simulink model "Quadruped_modelling"  (R2023b)
settings: Solver=VariableStepAuto  StartTime=0.0  StopTime=2.6  RelTol=1e-3
InitFcn:
  | robotParameters
undefined symbols (not defined in the file): foot_x, foot_y, foot_z, lower_leg_length, plane_x, plane_y, plane_z, torso_height, torso_length, torso_width, upper_leg_length, X, Y, Z
libraries: sm_lib x311, nesl_utility x41, walkingRobotUtils x4, sharedtransform x1
(part 9 of 9)

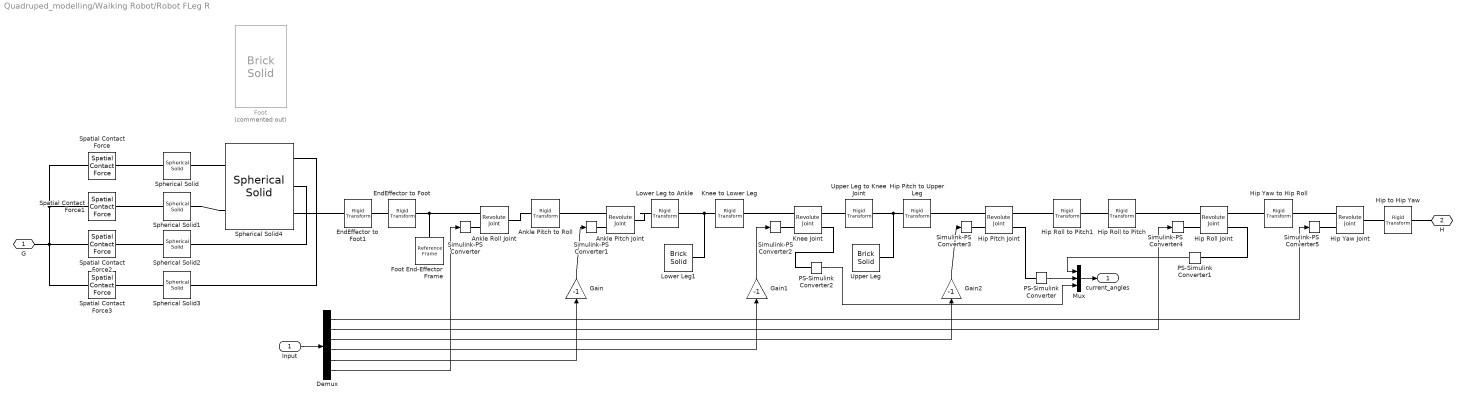
== system Quadruped_modelling/Walking Robot/Robot FLeg R ==
  Input : Inport
  Ankle Pitch Joint : sm_lib/Joints/Revolute Joint  JointMode=Normal  SenseConstraintForce=off  SenseConstraintForceX=off  SenseConstraintForceY=off  SenseConstraintForceZ=off  SenseConstraintTorque=off  SenseConstraintTorqueX=off  SenseConstraintTorqueY=off  SenseConstraintTorqueZ=off  SenseTotalForce=off  SenseTotalForceX=off  SenseTotalForceY=off  SenseTotalForceZ=off  SenseTotalTorque=off  SenseTotalTorqueX=off  SenseTotalTorqueY=off  SenseTotalTorqueZ=off  CompositeWrenchDir=FollowerOnBase  CompositeWrenchFrame=BaseFrame  EquilibriumPosition=0  EquilibriumPositionUnits=deg  SpringStiffness=0  SpringStiffnessUnits=N*m/deg  DampingCoefficient=1  DampingCoefficientUnits=N*m/(rad/s)  TorqueActuationMode=ComputedTorque  MotionActuationMode=InputMotion  SensePosition=off  SenseVelocity=off  SenseAcceleration=off  SenseTorqueForce=off  SenseLowerLimitTorqueForce=off  SenseUpperLimitTorqueForce=off  LowerLimitSpecify=on  LowerLimitBound=-pi/2  LowerLimitBoundUnits=rad  LowerLimitStiffness=100  LowerLimitStiffnessUnits=N*m/rad  LowerLimitDamping=10  LowerLimitDampingUnits=N*m/(rad/s)  LowerLimitTransitionRegionWidth=0.1  LowerLimitTransitionRegionWidthUnits=deg  UpperLimitSpecify=on  UpperLimitBound=pi/2  UpperLimitBoundUnits=rad  UpperLimitStiffness=100  UpperLimitStiffnessUnits=N*m/rad  UpperLimitDamping=10  UpperLimitDampingUnits=N*m/(rad/s)  UpperLimitTransitionRegionWidth=0.1  UpperLimitTransitionRegionWidthUnits=deg  PositionTargetSpecify=on  PositionTargetPriority=High  PositionTargetValue=0  PositionTargetValueUnits=rad  VelocityTargetSpecify=off  VelocityTargetPriority=High  VelocityTargetValue=0  VelocityTargetValueUnits=deg/s
  Ankle Pitch to Roll : sm_lib/Frames and Transforms/Rigid Transform  TranslationMethod=None  TranslationStandardOffset=0  TranslationStandardOffsetUnits=cm  TranslationStandardAxis=+Z  TranslationCartesianOffset=[0 0 upper_leg_length/2]  TranslationCartesianOffsetUnits=cm  TranslationROffset=0  TranslationROffsetUnits=m  TranslationZOffset=0  TranslationZOffsetUnits=m  TranslationThetaOffset=0  TranslationThetaOffsetUnits=deg  RotationMethod=StandardAxis  RotationAngleUnits=deg  RotationStandardAxis=+X  RotationAngle=90  RotationArbitraryAxis=[0 0 1]  FollAlignAxisA=+X  BaseAlignAxisA=+Y  FollAlignAxisB=+Y  BaseAlignAxisB=+Z  RotationSequenceAxes=FollowerAxes  RotationSequence=XYX  RotationSequenceAngles=[0 0 0]  RotationSequenceAnglesUnits=deg  RotationMatrix=[1 0 0; 0 1 0; 0 0 1]  Quaternion=[1 0 0 0]
  Ankle Roll Joint : sm_lib/Joints/Revolute Joint  JointMode=Normal  SenseConstraintForce=off  SenseConstraintForceX=off  SenseConstraintForceY=off  SenseConstraintForceZ=off  SenseConstraintTorque=off  SenseConstraintTorqueX=off  SenseConstraintTorqueY=off  SenseConstraintTorqueZ=off  SenseTotalForce=off  SenseTotalForceX=off  SenseTotalForceY=off  SenseTotalForceZ=off  SenseTotalTorque=off  SenseTotalTorqueX=off  SenseTotalTorqueY=off  SenseTotalTorqueZ=off  CompositeWrenchDir=FollowerOnBase  CompositeWrenchFrame=BaseFrame  EquilibriumPosition=0  EquilibriumPositionUnits=deg  SpringStiffness=0  SpringStiffnessUnits=N*m/deg  DampingCoefficient=1  DampingCoefficientUnits=N*m/(rad/s)  TorqueActuationMode=ComputedTorque  MotionActuationMode=InputMotion  SensePosition=off  SenseVelocity=off  SenseAcceleration=off  SenseTorqueForce=off  SenseLowerLimitTorqueForce=off  SenseUpperLimitTorqueForce=off  LowerLimitSpecify=on  LowerLimitBound=-pi/2  LowerLimitBoundUnits=rad  LowerLimitStiffness=100  LowerLimitStiffnessUnits=N*m/rad  LowerLimitDamping=10  LowerLimitDampingUnits=N*m/(rad/s)  LowerLimitTransitionRegionWidth=0.1  LowerLimitTransitionRegionWidthUnits=deg  UpperLimitSpecify=on  UpperLimitBound=pi/2  UpperLimitBoundUnits=rad  UpperLimitStiffness=100  UpperLimitStiffnessUnits=N*m/rad  UpperLimitDamping=10  UpperLimitDampingUnits=N*m/(rad/s)  UpperLimitTransitionRegionWidth=0.1  UpperLimitTransitionRegionWidthUnits=deg  PositionTargetSpecify=on  PositionTargetPriority=High  PositionTargetValue=0  PositionTargetValueUnits=rad  VelocityTargetSpecify=off  VelocityTargetPriority=High  VelocityTargetValue=0  VelocityTargetValueUnits=deg/s
  Demux : Demux  Outputs=6
  EndEffector to Foot : sm_lib/Frames and Transforms/Rigid Transform  TranslationMethod=None  TranslationStandardOffset=0  TranslationStandardOffsetUnits=cm  TranslationStandardAxis=+Z  TranslationCartesianOffset=[0 0 upper_leg_length/2]  TranslationCartesianOffsetUnits=cm  TranslationROffset=0  TranslationROffsetUnits=m  TranslationZOffset=0  TranslationZOffsetUnits=m  TranslationThetaOffset=0  TranslationThetaOffsetUnits=deg  RotationMethod=StandardAxis  RotationAngleUnits=deg  RotationStandardAxis=+Z  RotationAngle=-90  RotationArbitraryAxis=[0 0 1]  FollAlignAxisA=+X  BaseAlignAxisA=+Y  FollAlignAxisB=+Y  BaseAlignAxisB=+Z  RotationSequenceAxes=FollowerAxes  RotationSequence=XYX  RotationSequenceAngles=[0 0 0]  RotationSequenceAnglesUnits=deg  RotationMatrix=[1 0 0; 0 1 0; 0 0 1]  Quaternion=[1 0 0 0]
  EndEffector to Foot1 : sm_lib/Frames and Transforms/Rigid Transform  TranslationMethod=None  TranslationStandardOffset=0  TranslationStandardOffsetUnits=cm  TranslationStandardAxis=+Z  TranslationCartesianOffset=[0 0 upper_leg_length/2]  TranslationCartesianOffsetUnits=cm  TranslationROffset=0  TranslationROffsetUnits=m  TranslationZOffset=0  TranslationZOffsetUnits=m  TranslationThetaOffset=0  TranslationThetaOffsetUnits=deg  RotationMethod=StandardAxis  RotationAngleUnits=deg  RotationStandardAxis=+X  RotationAngle=180  RotationArbitraryAxis=[0 0 1]  FollAlignAxisA=+X  BaseAlignAxisA=+Y  FollAlignAxisB=+Y  BaseAlignAxisB=+Z  RotationSequenceAxes=FollowerAxes  RotationSequence=XYX  RotationSequenceAngles=[0 0 0]  RotationSequenceAnglesUnits=deg  RotationMatrix=[1 0 0; 0 1 0; 0 0 1]  Quaternion=[1 0 0 0]
  Foot : sm_lib/Body Elements/Brick Solid  Commented=on  GraphicAmbientColor=[0.15 0.15 0.15 1.0]  BasedOnType=Density  BrickDimensions=[foot_x foot_y foot_z]  BrickDimensionsUnits=m  CenterOfMass=[0 0 0]  CenterOfMassUnits=m  GraphicDiffuseColor=[0.5 0.5 0.5]  Density=200  DensityUnits=kg/(m^3)  DoExposeReferenceFrame=off  GraphicEmissiveColor=[0.0 0.0 0.0 1.0]  ExportEntireGeometry=off  SerializedFrames=<Frames><Frame><Id>Frame1</Id><Value><Name>F1</Name><Origin><Source>GeometricFeature</Source><FeatureName>+x -y curve</FeatureName></Origin><PrimaryAxis><DefinedDirection>+Z</DefinedDirection><Source>ReferenceFrame</Source><SourceDirection>+Z</SourceDirection><FeatureName></FeatureName></PrimaryAxis><SecondaryAxis><DefinedDirection>+X</DefinedDirection><Source>ReferenceFrame</Source><SourceDirection>+X</SourceDirection><FeatureName></FeatureName></SecondaryAxis></Value></Frame><Frame><Id>Frame2</Id><Value><Name>F2</Name><Origin><Source>GeometricFeature</Source><FeatureName>+x +y curve</FeatureName></Origin><PrimaryAxis><DefinedDirection>+Z</DefinedDirection><Source>ReferenceFrame</Source><SourceDirection>+Z</SourceDirection><FeatureName></FeatureName></PrimaryAxis><SecondaryAxis><DefinedDirection>+X</DefinedDirection><Source>ReferenceFrame</Source><SourceDirection>+X</SourceDirection><FeatureName></FeatureName></SecondaryAxis></Value></Frame><Frame><Id>Frame3</Id><Value><Name>F3</Name><Origin><Source>GeometricFeature</Source><FeatureName>-x -y curve</FeatureName></Origin><PrimaryAxis><DefinedDirection>+Z</DefinedDirection><Source>ReferenceFrame</Source><SourceDirection>+Z</SourceDirection><FeatureName></FeatureName></PrimaryAxis><SecondaryAxis><DefinedDirection>+X</DefinedDirection><Source>ReferenceFrame</Source><SourceDirection>+X</SourceDirection><FeatureName></FeatureName></SecondaryAxis></Value></Frame><Frame><Id>Frame4</Id><Value><Name>F4</Name><Origin><Source>GeometricFeature</Source><FeatureName>-x +y curve</FeatureName></Origin><PrimaryAxis><DefinedDirection>+Z</DefinedDirection><Source>ReferenceFrame</Source><SourceDirection>+Z</SourceDirection><FeatureName></FeatureName></PrimaryAxis><SecondaryAxis><DefinedDirection>+X</DefinedDirection><Source>ReferenceFrame</Source><SourceDirection>+X</SourceDirection><FeatureName></FeatureName></SecondaryAxis></Value></Frame><Frame><Id>Frame5</Id><Value><Name>A</Name><Origin><Source>GeometricFeature</Source><FeatureName>+z surface</FeatureName></Origin><PrimaryAxis><DefinedDirection>+Z</DefinedDirection><Source>ReferenceFrame</Source><SourceDirection>-Y</SourceDirection><FeatureName></FeatureName></PrimaryAxis><SecondaryAxis><DefinedDirection>+X</DefinedDirection><Source>ReferenceFrame</Source><SourceDirection>+X</SourceDirection><FeatureName></FeatureName></SecondaryAxis></Value></Frame></Frames>  MarkerShape=Sphere  MarkerSize=10  GraphicType=FromGeometry  InertiaType=CalculateFromGeometry  Mass=1  MassUnits=kg  MomentsOfInertia=[1 1 1]  MomentsOfInertiaUnits=kg*m^2  GraphicOpacity=1.0  ProductsOfInertia=[0 0 0]  ProductsOfInertiaUnits=kg*m^2  GraphicShininess=75  GraphicSpecularColor=[0.5 0.5 0.5 1.0]  GraphicVisPropType=SimpleVisualProperties
  Foot End-Effector Frame : sm_lib/Frames and Transforms/Reference Frame
  Gain : Gain  Gain=-1
  Gain1 : Gain  Gain=-1
  Gain2 : Gain  Gain=-1
  Hip Pitch Joint : sm_lib/Joints/Revolute Joint  JointMode=Normal  SenseConstraintForce=off  SenseConstraintForceX=off  SenseConstraintForceY=off  SenseConstraintForceZ=off  SenseConstraintTorque=off  SenseConstraintTorqueX=off  SenseConstraintTorqueY=off  SenseConstraintTorqueZ=off  SenseTotalForce=off  SenseTotalForceX=off  SenseTotalForceY=off  SenseTotalForceZ=off  SenseTotalTorque=off  SenseTotalTorqueX=off  SenseTotalTorqueY=off  SenseTotalTorqueZ=off  CompositeWrenchDir=FollowerOnBase  CompositeWrenchFrame=BaseFrame  EquilibriumPosition=0  EquilibriumPositionUnits=deg  SpringStiffness=0  SpringStiffnessUnits=N*m/deg  DampingCoefficient=1  DampingCoefficientUnits=N*m/(rad/s)  TorqueActuationMode=ComputedTorque  MotionActuationMode=InputMotion  SensePosition=on  SenseVelocity=off  SenseAcceleration=off  SenseTorqueForce=off  SenseLowerLimitTorqueForce=off  SenseUpperLimitTorqueForce=off  LowerLimitSpecify=on  LowerLimitBound=-pi/2  LowerLimitBoundUnits=rad  LowerLimitStiffness=100  LowerLimitStiffnessUnits=N*m/rad  LowerLimitDamping=10  LowerLimitDampingUnits=N*m/(rad/s)  LowerLimitTransitionRegionWidth=0.1  LowerLimitTransitionRegionWidthUnits=deg  UpperLimitSpecify=on  UpperLimitBound=pi/2  UpperLimitBoundUnits=rad  UpperLimitStiffness=100  UpperLimitStiffnessUnits=N*m/rad  UpperLimitDamping=10  UpperLimitDampingUnits=N*m/(rad/s)  UpperLimitTransitionRegionWidth=0.1  UpperLimitTransitionRegionWidthUnits=deg  PositionTargetSpecify=on  PositionTargetPriority=High  PositionTargetValue=0  PositionTargetValueUnits=rad  VelocityTargetSpecify=off  VelocityTargetPriority=High  VelocityTargetValue=0  VelocityTargetValueUnits=deg/s
  Hip Pitch to Upper Leg : sm_lib/Frames and Transforms/Rigid Transform  TranslationMethod=StandardAxis  TranslationStandardOffset=upper_leg_length/2  TranslationStandardOffsetUnits=m  TranslationStandardAxis=+X  TranslationCartesianOffset=[upper_leg_length/2 0 0]  TranslationCartesianOffsetUnits=m  TranslationROffset=0  TranslationROffsetUnits=m  TranslationZOffset=0  TranslationZOffsetUnits=m  TranslationThetaOffset=0  TranslationThetaOffsetUnits=deg  RotationMethod=StandardAxis  RotationAngleUnits=deg  RotationStandardAxis=+Y  RotationAngle=90  RotationArbitraryAxis=[0 0 1]  FollAlignAxisA=+X  BaseAlignAxisA=+Y  FollAlignAxisB=+Y  BaseAlignAxisB=+Z  RotationSequenceAxes=FollowerAxes  RotationSequence=XYX  RotationSequenceAngles=[0 0 0]  RotationSequenceAnglesUnits=deg  RotationMatrix=[1 0 0; 0 1 0; 0 0 1]  Quaternion=[1 0 0 0]
  Hip Roll Joint : sm_lib/Joints/Revolute Joint  JointMode=Normal  SenseConstraintForce=off  SenseConstraintForceX=off  SenseConstraintForceY=off  SenseConstraintForceZ=off  SenseConstraintTorque=off  SenseConstraintTorqueX=off  SenseConstraintTorqueY=off  SenseConstraintTorqueZ=off  SenseTotalForce=off  SenseTotalForceX=off  SenseTotalForceY=off  SenseTotalForceZ=off  SenseTotalTorque=off  SenseTotalTorqueX=off  SenseTotalTorqueY=off  SenseTotalTorqueZ=off  CompositeWrenchDir=FollowerOnBase  CompositeWrenchFrame=BaseFrame  EquilibriumPosition=0  EquilibriumPositionUnits=deg  SpringStiffness=0  SpringStiffnessUnits=N*m/deg  DampingCoefficient=1  DampingCoefficientUnits=N*m/(rad/s)  TorqueActuationMode=ComputedTorque  MotionActuationMode=InputMotion  SensePosition=on  SenseVelocity=off  SenseAcceleration=off  SenseTorqueForce=off  SenseLowerLimitTorqueForce=off  SenseUpperLimitTorqueForce=off  LowerLimitSpecify=on  LowerLimitBound=-pi/2  LowerLimitBoundUnits=rad  LowerLimitStiffness=100  LowerLimitStiffnessUnits=N*m/rad  LowerLimitDamping=10  LowerLimitDampingUnits=N*m/(rad/s)  LowerLimitTransitionRegionWidth=0.1  LowerLimitTransitionRegionWidthUnits=deg  UpperLimitSpecify=on  UpperLimitBound=pi/2  UpperLimitBoundUnits=rad  UpperLimitStiffness=100  UpperLimitStiffnessUnits=N*m/rad  UpperLimitDamping=10  UpperLimitDampingUnits=N*m/(rad/s)  UpperLimitTransitionRegionWidth=0.1  UpperLimitTransitionRegionWidthUnits=deg  PositionTargetSpecify=on  PositionTargetPriority=High  PositionTargetValue=0  PositionTargetValueUnits=rad  VelocityTargetSpecify=off  VelocityTargetPriority=High  VelocityTargetValue=0  VelocityTargetValueUnits=deg/s
  Hip Roll to Pitch : sm_lib/Frames and Transforms/Rigid Transform  TranslationMethod=None  TranslationStandardOffset=0  TranslationStandardOffsetUnits=cm  TranslationStandardAxis=+Z  TranslationCartesianOffset=[0 0 upper_leg_length/2]  TranslationCartesianOffsetUnits=cm  TranslationROffset=0  TranslationROffsetUnits=m  TranslationZOffset=0  TranslationZOffsetUnits=m  TranslationThetaOffset=0  TranslationThetaOffsetUnits=deg  RotationMethod=StandardAxis  RotationAngleUnits=deg  RotationStandardAxis=+Z  RotationAngle=-90  RotationArbitraryAxis=[0 0 1]  FollAlignAxisA=+X  BaseAlignAxisA=+Y  FollAlignAxisB=+Y  BaseAlignAxisB=+Z  RotationSequenceAxes=FollowerAxes  RotationSequence=XYX  RotationSequenceAngles=[0 0 0]  RotationSequenceAnglesUnits=deg  RotationMatrix=[1 0 0; 0 1 0; 0 0 1]  Quaternion=[1 0 0 0]
  Hip Roll to Pitch1 : sm_lib/Frames and Transforms/Rigid Transform  TranslationMethod=None  TranslationStandardOffset=0  TranslationStandardOffsetUnits=cm  TranslationStandardAxis=+Z  TranslationCartesianOffset=[0 0 upper_leg_length/2]  TranslationCartesianOffsetUnits=cm  TranslationROffset=0  TranslationROffsetUnits=m  TranslationZOffset=0  TranslationZOffsetUnits=m  TranslationThetaOffset=0  TranslationThetaOffsetUnits=deg  RotationMethod=StandardAxis  RotationAngleUnits=deg  RotationStandardAxis=+X  RotationAngle=-90  RotationArbitraryAxis=[0 0 1]  FollAlignAxisA=+X  BaseAlignAxisA=+Y  FollAlignAxisB=+Y  BaseAlignAxisB=+Z  RotationSequenceAxes=FollowerAxes  RotationSequence=XYX  RotationSequenceAngles=[0 0 0]  RotationSequenceAnglesUnits=deg  RotationMatrix=[1 0 0; 0 1 0; 0 0 1]  Quaternion=[1 0 0 0]
  Hip Yaw Joint : sm_lib/Joints/Revolute Joint  JointMode=Normal  SenseConstraintForce=off  SenseConstraintForceX=off  SenseConstraintForceY=off  SenseConstraintForceZ=off  SenseConstraintTorque=off  SenseConstraintTorqueX=off  SenseConstraintTorqueY=off  SenseConstraintTorqueZ=off  SenseTotalForce=off  SenseTotalForceX=off  SenseTotalForceY=off  SenseTotalForceZ=off  SenseTotalTorque=off  SenseTotalTorqueX=off  SenseTotalTorqueY=off  SenseTotalTorqueZ=off  CompositeWrenchDir=FollowerOnBase  CompositeWrenchFrame=BaseFrame  EquilibriumPosition=0  EquilibriumPositionUnits=deg  SpringStiffness=0  SpringStiffnessUnits=N*m/deg  DampingCoefficient=1  DampingCoefficientUnits=N*m/(rad/s)  TorqueActuationMode=ComputedTorque  MotionActuationMode=InputMotion  SensePosition=off  SenseVelocity=off  SenseAcceleration=off  SenseTorqueForce=off  SenseLowerLimitTorqueForce=off  SenseUpperLimitTorqueForce=off  LowerLimitSpecify=on  LowerLimitBound=-pi/2  LowerLimitBoundUnits=rad  LowerLimitStiffness=100  LowerLimitStiffnessUnits=N*m/rad  LowerLimitDamping=10  LowerLimitDampingUnits=N*m/(rad/s)  LowerLimitTransitionRegionWidth=0.1  LowerLimitTransitionRegionWidthUnits=deg  UpperLimitSpecify=on  UpperLimitBound=pi/2  UpperLimitBoundUnits=rad  UpperLimitStiffness=100  UpperLimitStiffnessUnits=N*m/rad  UpperLimitDamping=10  UpperLimitDampingUnits=N*m/(rad/s)  UpperLimitTransitionRegionWidth=0.1  UpperLimitTransitionRegionWidthUnits=deg  PositionTargetSpecify=on  PositionTargetPriority=High  PositionTargetValue=0  PositionTargetValueUnits=rad  VelocityTargetSpecify=off  VelocityTargetPriority=High  VelocityTargetValue=0  VelocityTargetValueUnits=deg/s
  Hip Yaw to Hip Roll : sm_lib/Frames and Transforms/Rigid Transform  TranslationMethod=None  TranslationStandardOffset=0  TranslationStandardOffsetUnits=cm  TranslationStandardAxis=+Z  TranslationCartesianOffset=[0 0 upper_leg_length/2]  TranslationCartesianOffsetUnits=cm  TranslationROffset=0  TranslationROffsetUnits=m  TranslationZOffset=0  TranslationZOffsetUnits=m  TranslationThetaOffset=0  TranslationThetaOffsetUnits=deg  RotationMethod=StandardAxis  RotationAngleUnits=deg  RotationStandardAxis=+X  RotationAngle=90  RotationArbitraryAxis=[0 0 1]  FollAlignAxisA=+X  BaseAlignAxisA=+Y  FollAlignAxisB=+Y  BaseAlignAxisB=+Z  RotationSequenceAxes=FollowerAxes  RotationSequence=XYX  RotationSequenceAngles=[0 0 0]  RotationSequenceAnglesUnits=deg  RotationMatrix=[1 0 0; 0 1 0; 0 0 1]  Quaternion=[1 0 0 0]
  Hip to Hip Yaw : sm_lib/Frames and Transforms/Rigid Transform  TranslationMethod=None  TranslationStandardOffset=0  TranslationStandardOffsetUnits=cm  TranslationStandardAxis=+Z  TranslationCartesianOffset=[0 0 upper_leg_length/2]  TranslationCartesianOffsetUnits=cm  TranslationROffset=0  TranslationROffsetUnits=m  TranslationZOffset=0  TranslationZOffsetUnits=m  TranslationThetaOffset=0  TranslationThetaOffsetUnits=deg  RotationMethod=StandardAxis  RotationAngleUnits=deg  RotationStandardAxis=+Z  RotationAngle=180  RotationArbitraryAxis=[0 0 1]  FollAlignAxisA=+X  BaseAlignAxisA=+Y  FollAlignAxisB=+Y  BaseAlignAxisB=+Z  RotationSequenceAxes=FollowerAxes  RotationSequence=XYX  RotationSequenceAngles=[0 0 0]  RotationSequenceAnglesUnits=deg  RotationMatrix=[1 0 0; 0 1 0; 0 0 1]  Quaternion=[1 0 0 0]
  Knee Joint : sm_lib/Joints/Revolute Joint  JointMode=Normal  SenseConstraintForce=off  SenseConstraintForceX=off  SenseConstraintForceY=off  SenseConstraintForceZ=off  SenseConstraintTorque=off  SenseConstraintTorqueX=off  SenseConstraintTorqueY=off  SenseConstraintTorqueZ=off  SenseTotalForce=off  SenseTotalForceX=off  SenseTotalForceY=off  SenseTotalForceZ=off  SenseTotalTorque=off  SenseTotalTorqueX=off  SenseTotalTorqueY=off  SenseTotalTorqueZ=off  CompositeWrenchDir=FollowerOnBase  CompositeWrenchFrame=BaseFrame  EquilibriumPosition=0  EquilibriumPositionUnits=deg  SpringStiffness=0  SpringStiffnessUnits=N*m/deg  DampingCoefficient=1  DampingCoefficientUnits=N*m/(rad/s)  TorqueActuationMode=ComputedTorque  MotionActuationMode=InputMotion  SensePosition=on  SenseVelocity=off  SenseAcceleration=off  SenseTorqueForce=off  SenseLowerLimitTorqueForce=off  SenseUpperLimitTorqueForce=off  LowerLimitSpecify=on  LowerLimitBound=-pi/2  LowerLimitBoundUnits=rad  LowerLimitStiffness=100  LowerLimitStiffnessUnits=N*m/rad  LowerLimitDamping=10  LowerLimitDampingUnits=N*m/(rad/s)  LowerLimitTransitionRegionWidth=0.1  LowerLimitTransitionRegionWidthUnits=deg  UpperLimitSpecify=on  UpperLimitBound=pi/2  UpperLimitBoundUnits=rad  UpperLimitStiffness=100  UpperLimitStiffnessUnits=N*m/rad  UpperLimitDamping=10  UpperLimitDampingUnits=N*m/(rad/s)  UpperLimitTransitionRegionWidth=0.1  UpperLimitTransitionRegionWidthUnits=deg  PositionTargetSpecify=on  PositionTargetPriority=High  PositionTargetValue=0  PositionTargetValueUnits=rad  VelocityTargetSpecify=off  VelocityTargetPriority=High  VelocityTargetValue=0  VelocityTargetValueUnits=deg/s
  Knee to Lower Leg : sm_lib/Frames and Transforms/Rigid Transform  TranslationMethod=StandardAxis  TranslationStandardOffset=lower_leg_length/2  TranslationStandardOffsetUnits=m  TranslationStandardAxis=+X  TranslationCartesianOffset=[upper_leg_length/2 0 0]  TranslationCartesianOffsetUnits=m  TranslationROffset=0  TranslationROffsetUnits=m  TranslationZOffset=0  TranslationZOffsetUnits=m  TranslationThetaOffset=0  TranslationThetaOffsetUnits=deg  RotationMethod=StandardAxis  RotationAngleUnits=deg  RotationStandardAxis=+Y  RotationAngle=90  RotationArbitraryAxis=[0 0 1]  FollAlignAxisA=+X  BaseAlignAxisA=+Y  FollAlignAxisB=+Y  BaseAlignAxisB=+Z  RotationSequenceAxes=FollowerAxes  RotationSequence=XYX  RotationSequenceAngles=[0 0 0]  RotationSequenceAnglesUnits=deg  RotationMatrix=[1 0 0; 0 1 0; 0 0 1]  Quaternion=[1 0 0 0]
  Lower Leg to Ankle : sm_lib/Frames and Transforms/Rigid Transform  TranslationMethod=StandardAxis  TranslationStandardOffset=lower_leg_length/2  TranslationStandardOffsetUnits=m  TranslationStandardAxis=+Z  TranslationCartesianOffset=[upper_leg_length/2 0 0]  TranslationCartesianOffsetUnits=m  TranslationROffset=0  TranslationROffsetUnits=m  TranslationZOffset=0  TranslationZOffsetUnits=m  TranslationThetaOffset=0  TranslationThetaOffsetUnits=deg  RotationMethod=StandardAxis  RotationAngleUnits=deg  RotationStandardAxis=+Y  RotationAngle=-90  RotationArbitraryAxis=[0 0 1]  FollAlignAxisA=+X  BaseAlignAxisA=+Y  FollAlignAxisB=+Y  BaseAlignAxisB=+Z  RotationSequenceAxes=FollowerAxes  RotationSequence=XYX  RotationSequenceAngles=[0 0 0]  RotationSequenceAnglesUnits=deg  RotationMatrix=[1 0 0; 0 1 0; 0 0 1]  Quaternion=[1 0 0 0]
  Lower Leg1 : sm_lib/Body Elements/Brick Solid  GraphicAmbientColor=[0.15 0.15 0.15 1.0]  BasedOnType=Density  BrickDimensions=[0.08 0.08 0.25]  BrickDimensionsUnits=m  CenterOfMass=[0 0 0]  CenterOfMassUnits=m  GraphicDiffuseColor=[0.5 0.5 0.5]  Density=200  DensityUnits=kg/m^3  DoExposeReferenceFrame=on  GraphicEmissiveColor=[0.0 0.0 0.0 1.0]  ExportEntireGeometry=off  SerializedFrames=<Frames/>  MarkerShape=Sphere  MarkerSize=10  GraphicType=FromGeometry  InertiaType=CalculateFromGeometry  Mass=1  MassUnits=kg  MomentsOfInertia=[1 1 1]  MomentsOfInertiaUnits=kg*m^2  GraphicOpacity=1.0  ProductsOfInertia=[0 0 0]  ProductsOfInertiaUnits=kg*m^2  GraphicShininess=75  GraphicSpecularColor=[0.5 0.5 0.5 1.0]  GraphicVisPropType=SimpleVisualProperties
  Mux : Mux  Inputs=3
  PS-Simulink Converter : nesl_utility/PS-Simulink Converter  PhysicalDomain=network_engine_domain  SubClassName=ps_output  LeftPortType=input  RightPortType=output  PseudoPeriodic=off  Frequencies=[]  VectorFormat=inherit  Unit=inherit  AffineConversion=off
  PS-Simulink Converter1 : nesl_utility/PS-Simulink Converter  PhysicalDomain=network_engine_domain  SubClassName=ps_output  LeftPortType=input  RightPortType=output  PseudoPeriodic=off  Frequencies=[]  VectorFormat=inherit  Unit=inherit  AffineConversion=off
  PS-Simulink Converter2 : nesl_utility/PS-Simulink Converter  PhysicalDomain=network_engine_domain  SubClassName=ps_output  LeftPortType=input  RightPortType=output  PseudoPeriodic=off  Frequencies=[]  VectorFormat=inherit  Unit=inherit  AffineConversion=off
  Simulink-PS Converter{,1..5} (6 alike) : nesl_utility/Simulink-PS Converter  PhysicalDomain=network_engine_domain  SubClassName=ps_input  LeftPortType=input  RightPortType=output  PseudoPeriodic=off  Frequencies=[]  NoiseDistribution=none  NoiseParameters=[]  Unit=rad  AffineConversion=off  FilteringAndDerivatives=filter  SimscapeFilterOrder=2  InputFilterTimeConstant=motion_time_constant  UdotUserProvided=2
  Spatial Contact Force{,1..3} (4 alike) : sm_lib/Forces and Torques/Spatial Contact Force  SenseContactBaseRotation=off  SenseContactBaseTranslation=off  CoefficientOfDynamicFriction=mu_k  CoefficientOfStaticFriction=mu_s  NormalDamping=contact_damping  NormalDampingUnits=N/(m/s)  SenseContactSignal=off  NormalStiffness=contact_stiffness  NormalStiffnessUnits=N/m  FrictionalCriticalVelocity=mu_vth  FrictionalCriticalVelocityUnits=m/s  ZeroCrossDetectContactStartAndEnd=off  SenseContactFollowerRotation=off  SenseContactFollowerTranslation=off  FrictionType=SmoothStickSlip  SenseFrictionalForceMagnitude=off  SenseNormalForceMagnitude=off  NormalForceType=SmoothSpringDamper  SenseNormalVelocity=off  SensePenetrationDepth=off  SenseSeparationDistance=off  SenseTangentialVelocity=off  NormalTransitionRegionWidth=1e-4  NormalTransitionRegionWidthUnits=m
  Spherical Solid{,1..3} (4 alike) : sm_lib/Body Elements/Spherical Solid  GraphicAmbientColor=[0.15 0.15 0.15 1.0]  BasedOnType=Mass  CenterOfMass=[0 0 0]  CenterOfMassUnits=m  GraphicDiffuseColor=[0.5 0.5 0.5]  Density=1000  DensityUnits=kg/m^3  DoExposeReferenceFrame=on  GraphicEmissiveColor=[0.0 0.0 0.0 1.0]  ExportEntireGeometry=on  SerializedExposedGeometries=<ExposedGeometries><ExposedGeometry><RawGeometryId>entire</RawGeometryId><ExposedGeometryId>G</ExposedGeometryId></ExposedGeometry></ExposedGeometries>  SerializedFrames=<Frames/>  MarkerShape=Sphere  MarkerSize=10  GraphicType=FromGeometry  InertiaType=CalculateFromGeometry  Mass=1  MassUnits=g  MomentsOfInertia=[1 1 1]  MomentsOfInertiaUnits=kg*m^2  GraphicOpacity=1.0  ProductsOfInertia=[0 0 0]  ProductsOfInertiaUnits=kg*m^2  GraphicShininess=75  GraphicSpecularColor=[0.5 0.5 0.5 1.0]  SphereRadius=foot_z/2  SphereRadiusUnits=m  GraphicVisPropType=SimpleVisualProperties
  Spherical Solid4 : sm_lib/Body Elements/Spherical Solid  GraphicAmbientColor=[0.15 0.15 0.15 1.0]  BasedOnType=Density  CenterOfMass=[0 0 0]  CenterOfMassUnits=m  GraphicDiffuseColor=[0.5 0.5 0.5]  Density=1000  DensityUnits=kg/m^3  DoExposeReferenceFrame=off  GraphicEmissiveColor=[0.0 0.0 0.0 1.0]  ExportEntireGeometry=off  SerializedExposedGeometries=<exposedGeometries/>  SerializedFrames=<Frames><Frame><Id>Frame1</Id><Value><Name>F1</Name><Origin><Source>ReferenceFrame</Source><FeatureName></FeatureName></Origin><PrimaryAxis><DefinedDirection>+Z</DefinedDirection><Source>ReferenceFrame</Source><SourceDirection>+Z</SourceDirection><FeatureName></FeatureName></PrimaryAxis><SecondaryAxis><DefinedDirection>+X</DefinedDirection><Source>ReferenceFrame</Source><SourceDirection>+X</SourceDirection><FeatureName></FeatureName></SecondaryAxis></Value></Frame><Frame><Id>Frame2</Id><Value><Name>F2</Name><Origin><Source>ReferenceFrame</Source><FeatureName></FeatureName></Origin><PrimaryAxis><DefinedDirection>+Z</DefinedDirection><Source>ReferenceFrame</Source><SourceDirection>+Z</SourceDirection><FeatureName></FeatureName></PrimaryAxis><SecondaryAxis><DefinedDirection>+X</DefinedDirection><Source>ReferenceFrame</Source><SourceDirection>+X</SourceDirection><FeatureName></FeatureName></SecondaryAxis></Value></Frame><Frame><Id>Frame3</Id><Value><Name>F3</Name><Origin><Source>ReferenceFrame</Source><FeatureName></FeatureName></Origin><PrimaryAxis><DefinedDirection>+Z</DefinedDirection><Source>ReferenceFrame</Source><SourceDirection>+Z</SourceDirection><FeatureName></FeatureName></PrimaryAxis><SecondaryAxis><DefinedDirection>+X</DefinedDirection><Source>ReferenceFrame</Source><SourceDirection>+X</SourceDirection><FeatureName></FeatureName></SecondaryAxis></Value></Frame><Frame><Id>Frame4</Id><Value><Name>F4</Name><Origin><Source>ReferenceFrame</Source><FeatureName></FeatureName></Origin><PrimaryAxis><DefinedDirection>+Z</DefinedDirection><Source>ReferenceFrame</Source><SourceDirection>+Z</SourceDirection><FeatureName></FeatureName></PrimaryAxis><SecondaryAxis><DefinedDirection>+X</DefinedDirection><Source>ReferenceFrame</Source><SourceDirection>+X</SourceDirection><FeatureName></FeatureName></SecondaryAxis></Value></Frame><Frame><Id>Frame5</Id><Value><Name>A</Name><Origin><Source>ReferenceFrame</Source><FeatureName></FeatureName></Origin><PrimaryAxis><DefinedDirection>+Z</DefinedDirection><Source>ReferenceFrame</Source><SourceDirection>+Z</SourceDirection><FeatureName></FeatureName></PrimaryAxis><SecondaryAxis><DefinedDirection>+X</DefinedDirection><Source>ReferenceFrame</Source><SourceDirection>+X</SourceDirection><FeatureName></FeatureName></SecondaryAxis></Value></Frame></Frames>  MarkerShape=Sphere  MarkerSize=10  GraphicType=FromGeometry  InertiaType=CalculateFromGeometry  Mass=1  MassUnits=kg  MomentsOfInertia=[1 1 1]  MomentsOfInertiaUnits=kg*m^2  GraphicOpacity=1.0  ProductsOfInertia=[0 0 0]  ProductsOfInertiaUnits=kg*m^2  GraphicShininess=75  GraphicSpecularColor=[0.5 0.5 0.5 1.0]  SphereRadius=foot_radius  SphereRadiusUnits=m  GraphicVisPropType=SimpleVisualProperties
  Upper Leg : sm_lib/Body Elements/Brick Solid  GraphicAmbientColor=[0.15 0.15 0.15 1.0]  BasedOnType=Density  BrickDimensions=[0.08 0.08 0.27]  BrickDimensionsUnits=m  CenterOfMass=[0 0 0]  CenterOfMassUnits=m  GraphicDiffuseColor=[0.5 0.5 0.5]  Density=200  DensityUnits=kg/m^3  DoExposeReferenceFrame=on  GraphicEmissiveColor=[0.0 0.0 0.0 1.0]  ExportEntireGeometry=off  SerializedFrames=<Frames/>  MarkerShape=Sphere  MarkerSize=10  GraphicType=FromGeometry  InertiaType=CalculateFromGeometry  Mass=1  MassUnits=kg  MomentsOfInertia=[1 1 1]  MomentsOfInertiaUnits=kg*m^2  GraphicOpacity=1.0  ProductsOfInertia=[0 0 0]  ProductsOfInertiaUnits=kg*m^2  GraphicShininess=75  GraphicSpecularColor=[0.5 0.5 0.5 1.0]  GraphicVisPropType=SimpleVisualProperties
  Upper Leg to Knee Joint : sm_lib/Frames and Transforms/Rigid Transform  TranslationMethod=StandardAxis  TranslationStandardOffset=upper_leg_length/2  TranslationStandardOffsetUnits=m  TranslationStandardAxis=+Z  TranslationCartesianOffset=[upper_leg_length/2 0 0]  TranslationCartesianOffsetUnits=m  TranslationROffset=0  TranslationROffsetUnits=m  TranslationZOffset=0  TranslationZOffsetUnits=m  TranslationThetaOffset=0  TranslationThetaOffsetUnits=deg  RotationMethod=StandardAxis  RotationAngleUnits=deg  RotationStandardAxis=+Y  RotationAngle=-90  RotationArbitraryAxis=[0 0 1]  FollAlignAxisA=+X  BaseAlignAxisA=+Y  FollAlignAxisB=+Y  BaseAlignAxisB=+Z  RotationSequenceAxes=FollowerAxes  RotationSequence=XYX  RotationSequenceAngles=[0 0 0]  RotationSequenceAnglesUnits=deg  RotationMatrix=[1 0 0; 0 1 0; 0 0 1]  Quaternion=[1 0 0 0]
  G : PMIOPort  Side=Right
  H : PMIOPort  Port=2  Side=Right
  current_angles : Outport  VectorParamsAs1DForOutWhenUnconnected=off
  wires:
  Input/1 -> Demux/1
  Demux/6 -> Simulink-PS Converter/1
  Demux/5 -> Gain/1
  Demux/4 -> Gain1/1
  Demux/3 -> Gain2/1
  Demux/2 -> Simulink-PS Converter4/1
  Demux/1 -> Simulink-PS Converter5/1
  Gain/1 -> Simulink-PS Converter1/1
  Gain1/1 -> Simulink-PS Converter2/1
  Gain2/1 -> Simulink-PS Converter3/1
  PS-Simulink Converter/1 -> Mux/2
  Mux/1 -> current_angles/1
  PS-Simulink Converter1/1 -> Mux/1
  PS-Simulink Converter2/1 -> Mux/3
  connections:
  Knee Joint/LConn1 -- Knee to Lower Leg/LConn1
  Lower Leg to Ankle/RConn1 -- Ankle Pitch Joint/RConn1
  Knee Joint/RConn1 -- Upper Leg to Knee Joint/RConn1
  Hip to Hip Yaw/LConn1 -- H/RConn1
  Hip Roll to Pitch1/RConn1 -- Hip Pitch Joint/RConn1
  Hip Yaw Joint/LConn1 -- Hip Yaw to Hip Roll/LConn1
  Hip Yaw to Hip Roll/RConn1 -- Hip Roll Joint/RConn1
  Hip Roll Joint/LConn1 -- Hip Roll to Pitch/LConn1
  Hip Roll to Pitch1/LConn1 -- Hip Roll to Pitch/RConn1
  Hip Yaw Joint/RConn1 -- Hip to Hip Yaw/RConn1
  Hip Pitch Joint/LConn1 -- Hip Pitch to Upper Leg/LConn1
  Ankle Pitch Joint/LConn1 -- Ankle Pitch to Roll/LConn1
  EndEffector to Foot1/LConn1 -- EndEffector to Foot/RConn1
  EndEffector to Foot/LConn1 -- Ankle Roll Joint/LConn1 -- Foot End-Effector Frame/RConn1
  Ankle Pitch to Roll/RConn1 -- Ankle Roll Joint/RConn1
  Lower Leg to Ankle/LConn1 -- Knee to Lower Leg/RConn1 -- Lower Leg1/RConn1
  Hip Pitch to Upper Leg/RConn1 -- Upper Leg to Knee Joint/LConn1 -- Upper Leg/RConn1
  Simulink-PS Converter/RConn1 -- Ankle Roll Joint/LConn2
  Simulink-PS Converter1/RConn1 -- Ankle Pitch Joint/LConn2
  Simulink-PS Converter2/RConn1 -- Knee Joint/LConn2
  Simulink-PS Converter3/RConn1 -- Hip Pitch Joint/LConn2
  Simulink-PS Converter4/RConn1 -- Hip Roll Joint/LConn2
  Simulink-PS Converter5/RConn1 -- Hip Yaw Joint/LConn2
  EndEffector to Foot1/RConn1 -- Spherical Solid4/LConn3
  Spatial Contact Force1/LConn1 -- Spatial Contact Force3/LConn1 -- G/RConn1 -- Spatial Contact Force2/LConn1 -- Spatial Contact Force/LConn1
  Spherical Solid3/LConn1 -- Spatial Contact Force3/RConn1
  Spherical Solid1/LConn1 -- Spatial Contact Force1/RConn1
  Spherical Solid/LConn1 -- Spatial Contact Force/RConn1
  Spatial Contact Force2/RConn1 -- Spherical Solid2/LConn1
  Spherical Solid/RConn1 -- Spherical Solid4/RConn1
  Spherical Solid1/RConn1 -- Spherical Solid4/RConn2
  Spherical Solid2/RConn1 -- Spherical Solid4/LConn2
  Spherical Solid3/RConn1 -- Spherical Solid4/LConn1
  Hip Pitch Joint/RConn2 -- PS-Simulink Converter/LConn1
  Hip Roll Joint/RConn2 -- PS-Simulink Converter1/LConn1
  Knee Joint/RConn2 -- PS-Simulink Converter2/LConn1

== stateflow chart Quadruped_modelling/State Transitions ==
  state Initilisation
    next_state = 1;
  state Walking_Phase_fr_rl
    next_state = 2;
  state Stationary
    next_state = 4;
  state Walking_Phase_fl_rr
    next_state = 3;
  (default) -> Initilisation
  Initilisation -> Stationary : [ctrl_state==next_state]
  Stationary -> Walking_Phase_fr_rl : [mode >= 1 && ctrl_state == next_state]
  Walking_Phase_fl_rr -> Walking_Phase_fr_rl [order 2] : [ctrl_state == next_state]
  Walking_Phase_fr_rl -> (junction 49) [order 1] : [mode == 0]
  Walking_Phase_fr_rl -> Walking_Phase_fl_rr [order 2] : [ctrl_state == next_state]
  (junction 49) -> Stationary
  Walking_Phase_fl_rr -> (junction 49) [order 1] : [mode == 0]
  data: ctrl_state input =0; mode input =0; next_state output

== matlab function Quadruped_modelling/QuadCtrl ==
  settings: updateMethod=DISCRETE
  data: fl_ang input; tgt_ctrl_fl output; fr_ang input; rl_ang input; rr_ang input; tgt_ctrl_fr output; tgt_ctrl_rl output; tgt_ctrl_rr output; t input
function [tgt_ctrl_fl,tgt_ctrl_fr,tgt_ctrl_rl,tgt_ctrl_rr] = controller(fl_ang, fr_ang, rl_ang, rr_ang, t)
    
    if t < 1      % move joints into start configuration
        tgt_ctrl_fr = [0;0.131*(t);-1.19*(t)];
        tgt_ctrl_rl = [0;0.131*(t);-1.19*(t)];
        tgt_ctrl_fl = [0;1.0586*(t);-1.19*(t)];
        tgt_ctrl_rr = [0;1.0586*(t);-1.19*(t)];
        % tgt_ctrl_fl = [0;0;0];
        % tgt_ctrl_rr = [0;0;0];
    
    else                 % Walk cycle
        %% fr to joint
        [fr_tgt_ang_s,fr_tgt_ang_u,fr_tgt_ang_k] = inverse_kinematics_NOSHOULDER(t,1);
        tgt_ctrl_fr = [fr_tgt_ang_s;fr_tgt_ang_u;fr_tgt_ang_k];

        %% rl to joint
        [rl_tgt_ang_s,rl_tgt_ang_u,rl_tgt_ang_k] = inverse_kinematics_NOSHOULDER(t,1);
        tgt_ctrl_rl = [rl_tgt_ang_s;rl_tgt_ang_u;rl_tgt_ang_k];

        % tgt_ctrl_fl = [0;0;0];
        % tgt_ctrl_rr = [0;0;0];
        %% fl to joint
        [fl_tgt_ang_s,fl_tgt_ang_u,fl_tgt_ang_k] = inverse_kinematics_NOSHOULDER(t,0);
        tgt_ctrl_fl = [fl_tgt_ang_s;fl_tgt_ang_u;fl_tgt_ang_k];

        %% rr to joint
        [rr_tgt_ang_s,rr_tgt_ang_u,rr_tgt_ang_k] = inverse_kinematics_NOSHOULDER(t,0);
        tgt_ctrl_rr = [rr_tgt_ang_s;rr_tgt_ang_u;rr_tgt_ang_k];



        % %% fl to joint
        % [fl_tgt_ang_s,fl_tgt_ang_u,fl_tgt_ang_k] = inverse_kinematics_NOSHOULDER(t);
        % tgt_ctrl_fl = [fl_tgt_ang_s;fl_tgt_ang_u;fl_tgt_ang_k];
        % 
        % %% fr to joint
        % [fr_tgt_ang_s,fr_tgt_ang_u,fr_tgt_ang_k] = inverse_kinematics_NOSHOULDER(t);
        % tgt_ctrl_fr = [fr_tgt_ang_s;fr_tgt_ang_u;fr_tgt_ang_k];
        % 
        % %% rl to joint
        % [rl_tgt_ang_s,rl_tgt_ang_u,rl_tgt_ang_k] = inverse_kinematics_NOSHOULDER(t);
        % tgt_ctrl_rl = [rl_tgt_ang_s;rl_tgt_ang_u;rl_tgt_ang_k];
        % 
        % %% rr to joint
        % [rr_tgt_ang_s,rr_tgt_ang_u,rr_tgt_ang_k] = inverse_kinematics_NOSHOULDER(t);
        % tgt_ctrl_rr = [rr_tgt_ang_s;rr_tgt_ang_u;rr_tgt_ang_k];

    end
    

%% Inverse Kinematic Function
    function [q0, q1, q2] = inverse_kinematics_NOSHOULDER(t,pair)
        
        q0 = 0; %%% SHOULDER JOINT IGNORED FOR NOW
    
        if pair == 1
            xCoords = [-0.2 -0.15 -0.1 -0.05 0 0.05 0.1 0.15 0.2 0.1936 0.1732 0.1323 0 -0.1323 -0.1732 -0.1936];
            yCoords = [-0.4 -0.4 -0.4 -0.4 -0.4 -0.4 -0.4 -0.4 -0.4 -0.35 -0.3 -0.25 -0.2 -0.25 -0.3 -0.35];
        else
            xCoords = [0.2 0.1936 0.1732 0.1323 0 -0.1323 -0.1732 -0.1936 -0.2 -0.15 -0.1 -0.05 0 0.05 0.1 0.15];
            yCoords = [-0.4 -0.35 -0.3 -0.25 -0.2 -0.25 -0.3 -0.35 -0.4 -0.4 -0.4 -0.4 -0.4 -0.4 -0.4 -0.4 ];
        end

        % Stage timing
        currentStage = floor(t*10) - 4;
        nextStage = currentStage + 1;
        stageProgress = ( (floor(t*1000) - 1000)/100 ) - (currentStage-1);
        

        if nextStage > 16
            nextStage = 1;
        end

        differenceX = xCoords(nextStage) - xCoords(currentStage);
        differenceY = yCoords(nextStage) - yCoords(currentStage);

        currentXCoord = differenceX*stageProgress + xCoords(currentStage);
        currentYCoord = differenceY*stageProgress + yCoords(currentStage);
    
        q2 = acos((currentXCoord^2 + currentYCoord^2 - 0.27^2 - 0.27^2)/(2*0.27*0.27));
        q1 = ( atan(currentYCoord/currentXCoord) + atan((0.27*sin(q2))/(0.27 + 0.27*cos(q2))) );
        q2 = -q2;
        if pair == 0
            q1 = -q1 + pi/4;
        end
        if currentXCoord < 0
            q1 = q1 - pi/2;
        end
        
    end


end




% %unpack sensing_info
% body_vx = sensing_info(4);
% body_vy = sensing_info(5);
% 
% % distance from center of mass to shoulder
% fl_offset = [torso_width/2;torso_length/2+leg_width/2;0];
% fr_offset = [torso_width/2;-torso_length/2-leg_width/2;0];
% rl_offset = [torso_width/2;torso_length/2+leg_width/2;0];
% rr_offset = [torso_width/2;-torso_length/2-leg_width/2;0];
% 
% %decide state and state transition helpers
% persistent state;
% persistent timer;
% persistent timer2;
% if isempty(state)
%     state = 0;
% end
% if isempty(timer)
%     timer = 0;
% end
% if isempty(timer2)
%     timer2 = 0;
% end
% 
% % init variables
%            % fl fr rl rr
% has_u_ctrl = [1 1 1 1];
% normal_virtual_leg1 = [0;0;planner.stand_height];
% normal_virtual_leg2 = [0;0;planner.stand_height];
% move_fl_end_effector = normal_virtual_leg1;
% move_rr_end_effector = normal_virtual_leg1;
% move_fr_end_effector = normal_virtual_leg2;
% move_rl_end_effector = normal_virtual_leg2;
% 
% % turning on spot mechanic
% isTurning = mode == 2 || mode == 3;
% %{
% if isTurning
%     leg_a_coef = 1; % -1/3
%     leg_b_coef = 1;
% else
%     leg_a_coef = 1;
%     leg_b_coef = 1;
% end
% %}
% leg_a_coef = 1;
% leg_b_coef = 1;
% 
% % state machine
% 
% if state == 0 % standby state
%     % in this state, just do nothing, but use time to make sure that all
%     % feet stands on the ground
% 
%     if contact_state(1) == 1 && contact_state(2) == 1 && contact_state(3) == 1 && contact_state(4) == 1
%         %all foot on ground
%         if abs(body_vx) < planner.state0_vel_thres 
%             timer = timer + 1;
%         else
%             timer = 0;
%         end
%         if timer > planner.state0_trans_thres 
%             state = 1;
%             timer = 0;
%         end
%     end
% elseif state == 1 % swing whole body to get a inital velocity
%     timer2 = timer2 + 1;
%     move_theta = planner.state0_swing_ang*sin(2*pi/planner.state0_swing_T*timer2);
%     move_leg_Rx = [cos(move_theta) 0 sin(move_theta);
%         0 1 0;
%         -sin(move_theta) 0 cos(move_theta)];
%     tgt_virtual_leg1_b = move_leg_Rx*normal_virtual_leg1;
%     tgt_virtual_leg2_b = move_leg_Rx*normal_virtual_leg2;
%     move_fl_end_effector = tgt_virtual_leg1_b;
%     move_rr_end_effector = tgt_virtual_leg1_b;
%     move_fr_end_effector = tgt_virtual_leg2_b;
%     move_rl_end_effector = tgt_virtual_leg2_b;
% 
%     if body_vx > planner.state12_trans_speed
%         timer = timer + 1;
%     else
%         timer = 0;
%     end
%     if timer > 40  %(keep a velocity larger than 0.2 for 0.1s)
%         state = next_state;
%         timer = 0;
%         timer2 = 0;
%     end
% 
% elseif state == 2 % stance virtual leg1, swing virtual leg2
%     timer2 = timer2 + 1;
%     if timer2 > planner.leg_swing_time %(0.5s finish movement)
%         timer2 = planner.leg_swing_time;
%     end
%     % stance leg no u control but need to balance the body
%                % fl fr rl rr
%     has_u_ctrl = [0 1 1 0];
%     t = timer2/planner.leg_swing_time;
% %     stance_length_coeff = 0.95+0.05*(timer2/planner.leg_swing_time);
%     stance_length_coeff = 0.2*t^2 - 0.2*t + 1;
%     tgt_virtual_leg1_b = stance_length_coeff*normal_virtual_leg1;
%     move_fl_end_effector = tgt_virtual_leg1_b;
%     move_rr_end_effector = tgt_virtual_leg1_b;
% 
% 
%     % swing leg must consider body angle 
% %     move_theta = -11/180*pi*(t);
%     length_coeff = 0.8*t^2-0.8*t+1;
%     % move leg in x direction
%     move_theta = get_move_angle(length_coeff*normal_virtual_leg2,body_vx, planner.tgt_body_vx, planner);
% 
%     move_leg_Rx = [cos(move_theta) 0 sin(move_theta);
%         0 1 0;
%         -sin(move_theta) 0 cos(move_theta)];
%     move_leg_Rx2 = [cos(move_theta) 0 sin(move_theta);
%         0 1 0;
%         -sin(move_theta) 0 cos(move_theta)];
%     tgt_virtual_leg2_a = length_coeff*move_leg_Rx2*normal_virtual_leg2;
%     tgt_virtual_leg2_b = length_coeff*move_leg_Rx*normal_virtual_leg2;
% 
%     % move leg in y direction
%     sagittal_angle = get_sagittal_angle(tgt_virtual_leg2_b,body_R, body_vy, planner);
%     move_leg_Ry =[1 0 0;
%                  0 cos(sagittal_angle) -sin(sagittal_angle);
%                  0 sin(sagittal_angle) cos(sagittal_angle)];
%     tgt_virtual_leg2_b = move_leg_Ry*tgt_virtual_leg2_b;
%     tgt_virtual_leg2_a = move_leg_Ry*tgt_virtual_leg2_a;
% 
% 
%     move_fr_end_effector = body_R'*(tgt_virtual_leg2_b+fr_offset)-fr_offset;
%     if norm(move_fr_end_effector) > body.max_stretch
%         move_fr_end_effector = move_fr_end_effector/norm(move_fr_end_effector)*body.max_stretch;
%     end
%     move_rl_end_effector = body_R'*(tgt_virtual_leg2_a+rl_offset)-rl_offset;
%     if norm(move_rl_end_effector) > body.max_stretch
%         move_rl_end_effector = move_rl_end_effector/norm(move_rl_end_effector)*body.max_stretch;
%     end
% 
%     % state transition
% %     if timer2 == planner.leg_swing_time
%     if timer2 > 0.5*planner.leg_swing_time && contact_state(2) == 1 && contact_state(3) == 1
%         timer = timer + 1;
%     else
%         timer = 0;
%     end
%     if timer > 5   % to be determined
%         state = next_state;
%         timer = 0;
%         timer2 = 0;
%     end
% 
% elseif state == 3 % swing virtual leg1, stance virtual leg2
%     timer2 = timer2 + 1;
%     if timer2 > planner.leg_swing_time %(0.5s finish movement)
%         timer2 = planner.leg_swing_time;
%     end
%     % stance leg no u control but need to balance the body
%                % fl fr rl rr
%     has_u_ctrl = [1 0 0 1];
% %     stance_length_coeff = 0.95+0.05*(timer2/planner.leg_swing_time);
%     t = timer2/planner.leg_swing_time;
%     stance_length_coeff = 0.2*t^2 - 0.2*t + 1;
%     tgt_virtual_leg2_b = stance_length_coeff*normal_virtual_leg2;
%     move_fr_end_effector = tgt_virtual_leg2_b;
%     move_rl_end_effector = tgt_virtual_leg2_b;
% 
%     % swing leg must consider body angle 
%     % theta is a function of forward velocity 
% %     move_theta = -11/180*pi*(t);
%     length_coeff = 0.8*t^2-0.8*t+1;
%     move_theta = get_move_angle(length_coeff*normal_virtual_leg1,body_vx, planner.tgt_body_vx, planner);
%     move_leg_Rx = [cos(move_theta*(1-2*isTurning)) 0 sin(move_theta*(1-2*isTurning));
%         0 1 0;
%         -sin(move_theta*(1-2*isTurning)) 0 cos(move_theta*(1-2*isTurning))];
%     move_leg_Rx2 = [cos(move_theta*(1-2*isTurning)) 0 sin(move_theta*(1-2*isTurning));
%         0 1 0;
%         -sin(move_theta*(1-2*isTurning)) 0 cos(move_theta*(1-2*isTurning))];
%     tgt_virtual_leg1_a = length_coeff*move_leg_Rx2*normal_virtual_leg1;
%     tgt_virtual_leg1_b = length_coeff*move_leg_Rx*normal_virtual_leg1;
% 
%     % move leg in y direction
%     sagittal_angle = get_sagittal_angle(tgt_virtual_leg1_b,body_R, body_vy, planner);
%     move_leg_Ry =[1 0 0;
%                  0 cos(sagittal_angle) -sin(sagittal_angle);
%                  0 sin(sagittal_angle) cos(sagittal_angle)];
%     tgt_virtual_leg1_b = move_leg_Ry*tgt_virtual_leg1_b;
%     tgt_virtual_leg1_a = move_leg_Ry*tgt_virtual_leg1_a;
% 
%     move_fl_end_effector = body_R'*(tgt_virtual_leg1_b+fl_offset)-fl_offset;
%     if norm(move_fl_end_effector) > body.max_stretch
%         move_fl_end_effector = move_fl_end_effector/norm(move_fl_end_effector)*body.max_stretch;
%     end
%     move_rr_end_effector = body_R'*(tgt_virtual_leg1_a+rr_offset)-rr_offset;
%     if norm(move_rr_end_effector) > body.max_stretch
%         move_rr_end_effector = move_rr_end_effector/norm(move_rr_end_effector)*body.max_stretch;
%     end
% 
%     % state transition
% %     if timer2 == planner.leg_swing_time
%     if timer2 > 0.5*planner.leg_swing_time && contact_state(1) == 1 && contact_state(4) == 1
%         timer = timer + 1;
%     else
%         timer = 0;
%     end
%     if timer > 5   % to be determined
%         state = next_state;
%         timer = 0;
%         timer2 = 0;
%     end
% elseif state == 4 % stabalisation
%     timer2 = timer2 + 1;
%     move_theta = planner.state0_swing_ang*sin(2*pi/planner.state0_swing_T*timer2);
%     move_leg_Rx = [cos(move_theta) 0 sin(move_theta);
%         0 1 0;
%         -sin(move_theta) 0 cos(move_theta)];
%     tgt_virtual_leg1_b = move_leg_Rx*normal_virtual_leg1;
%     tgt_virtual_leg2_b = move_leg_Rx*normal_virtual_leg2;
%     move_fl_end_effector = tgt_virtual_leg1_b;
%     move_rr_end_effector = tgt_virtual_leg1_b;
%     move_fr_end_effector = tgt_virtual_leg2_b;
%     move_rl_end_effector = tgt_virtual_leg2_b;
% 
%     timer = timer + 1;
%     if timer > 40  %(keep a velocity larger than 0.2 for 0.1s)
%         state = next_state;
%         timer = 0;
%         timer2 = 0;
%     end
% end
% 
% %% fl to joint
% [inv_s,inv_u,inv_k] = inverse_kinematics(move_fl_end_effector, body);
% fl_tgt_ang_s = inv_s; 
% fl_tgt_ang_u = inv_u;       
% fl_tgt_ang_k = inv_k; 
% tgt_ctrl_fl = [fl_tgt_ang_s;fl_tgt_ang_u;fl_tgt_ang_k;has_u_ctrl(1)];
% 
% %% fr to joint
% [inv_s,inv_u,inv_k] = inverse_kinematics(move_fr_end_effector, body);
% fr_tgt_ang_s = inv_s;
% fr_tgt_ang_u = inv_u;
% fr_tgt_ang_k = inv_k;
% tgt_ctrl_fr = [fr_tgt_ang_s;fr_tgt_ang_u;fr_tgt_ang_k;has_u_ctrl(2)];
% 
% %% rl to joint
% [inv_s,inv_u,inv_k] = inverse_kinematics(move_rl_end_effector, body);
% rl_tgt_ang_s = inv_s;
% rl_tgt_ang_u = inv_u;
% rl_tgt_ang_k = inv_k;
% tgt_ctrl_rl = [rl_tgt_ang_s;rl_tgt_ang_u;rl_tgt_ang_k;has_u_ctrl(3)];
% 
% %% rr to joint
% [inv_s,inv_u,inv_k] = inverse_kinematics(move_rr_end_effector, body);
% rr_tgt_ang_s = inv_s;
% rr_tgt_ang_u = inv_u;
% rr_tgt_ang_k = inv_k; 
% tgt_ctrl_rr = [rr_tgt_ang_s;rr_tgt_ang_u;rr_tgt_ang_k;has_u_ctrl(4)];
% 
% ctrl_state = state;
% debug = timer;
% 
% end
% 
% function move_angle = get_move_angle(virtual_leg,body_vx, tgt_body_vx, planner)
% 
%     distance = body_vx* planner.Ts/2 + planner.Kv*(tgt_body_vx-body_vx);
% 
%     if distance > 0.5*norm(virtual_leg)
%         distance = 0.5*norm(virtual_leg);
%     elseif distance < -0.5*norm(virtual_leg)
%         distance = -0.5*norm(virtual_leg);
%     end
% 
%     move_angle = asin(distance/norm(virtual_leg));
%     if move_angle > 20/180*pi
%         move_angle = 20/180*pi;
%     elseif move_angle < -20/180*pi
%         move_angle = -20/180*pi;
%     end
% 
% end
% 
% function move_angle = get_sagittal_angle(virtual_leg,body_R, body_vy, planner)
% 
%     distance = body_vy* planner.y_Ts/2 + planner.y_Kv*(0-body_vy);  
% 
%     if distance > 0.5*norm(virtual_leg)
%         distance = 0.5*norm(virtual_leg);
%     elseif distance < -0.5*norm(virtual_leg)
%         distance = -0.5*norm(virtual_leg);
%     end
% 
%     move_angle = asin(distance/norm(virtual_leg));
%     if move_angle > 20/180*pi
%         move_angle = 20/180*pi;
%     elseif move_angle < -20/180*pi
%         move_angle = -20/180*pi;
%     end
% 
% end
